simulink model "sim_test_observer"  (R2015b)
settings: Solver=VariableStepAuto  StartTime=0.0  StopTime=100  RelTol=1e-3
libraries: cstblocks x4
settings Model: Creator=lbromo12  LastModifiedBy=alvaro

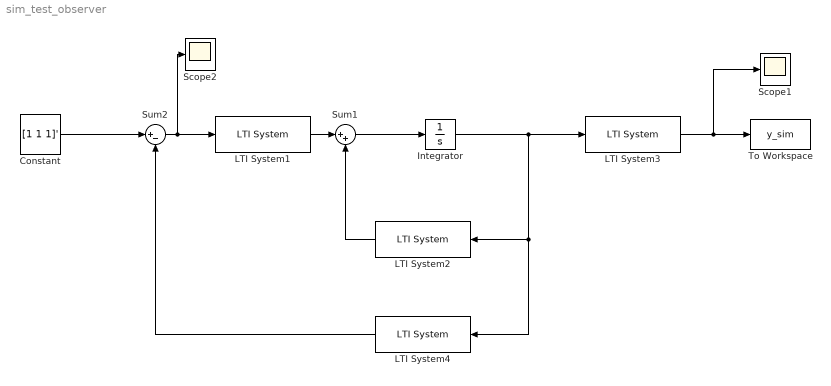
== system sim_test_observer ==
  Constant : Constant  Value=[1 1 1]'
  Integrator : Integrator
  LTI System1 : cstblocks/LTI System  sys=B  IC=[]
  LTI System2 : cstblocks/LTI System  sys=A  IC=[]
  LTI System3 : cstblocks/LTI System  sys=C  IC=[]
  LTI System4 : cstblocks/LTI System  sys=K  IC=[]
  Scope1 : Scope
  Scope2 : Scope
  Sum1 : Sum  Inputs=|++
  Sum2 : Sum  Inputs=|+-
  To Workspace : ToWorkspace  VariableName=y_sim  SaveFormat=Timeseries  SampleTime=-1
  wires:
  LTI System2/1 -> Sum1/2
  LTI System1/1 -> Sum1/1
  Sum1/1 -> Integrator/1
  LTI System3/1 -> Scope1/1, To Workspace/1
  Integrator/1 -> LTI System3/1, LTI System2/1, LTI System4/1
  LTI System4/1 -> Sum2/2
  Sum2/1 -> Scope2/1, LTI System1/1
  Constant/1 -> Sum2/1
